simulink model "z6_backup"  (R2016b)
settings: Solver=VariableStepAuto  StartTime=0.0  StopTime=10.0  RelTol=1e-3
values from neighbouring files (symbols this model uses):
  K = acker(A, B, p)    [z6.m]    (also in z7.m; z8.m)
  x0 = [0.1 0.1 0.1]    [z3.m]    (also in z6.m = [-1 2 1]; z7.m = [0 0 0]; z8.m = [-1 2 1])
settings Model: Creator=E7440  LastModifiedBy=E7440

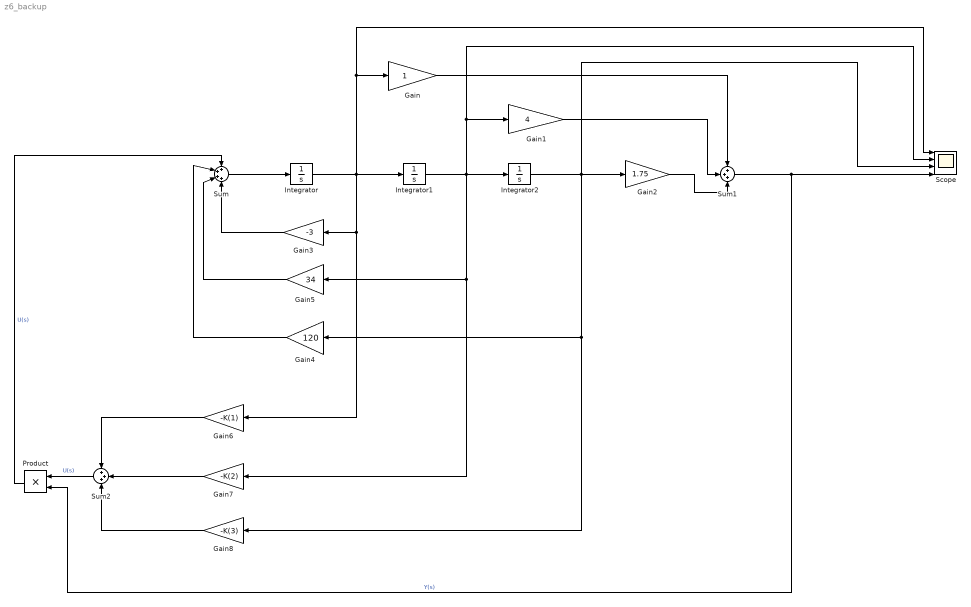
== system z6_backup ==
  Gain : Gain
  Gain1 : Gain  Gain=4
  Gain2 : Gain  Gain=1.75
  Gain3 : Gain  Gain=-3
  Gain4 : Gain  Gain=120
  Gain5 : Gain  Gain=34
  Gain6 : Gain  Gain=-K(1)
  Gain7 : Gain  Gain=-K(2)
  Gain8 : Gain  Gain=-K(3)
  Integrator : Integrator  InitialCondition=x0(1)
  Integrator1 : Integrator  InitialCondition=x0(2)
  Integrator2 : Integrator  InitialCondition=x0(3)
  Product : Product
  Scope : Scope  NumInputPorts=4
  Sum : Sum  Inputs=++++
  Sum1 : Sum  Inputs=+++
  Sum2 : Sum  Inputs=3
  wires:
  Product/1 -> Sum/1  "U(s)"
  Sum/1 -> Integrator/1
  Gain2/1 -> Sum1/3
  Gain1/1 -> Sum1/2
  Gain/1 -> Sum1/1
  Integrator2/1 -> Scope/3, Gain8/1, Gain4/1, Gain2/1
  Integrator/1 -> Integrator1/1, Gain6/1, Gain3/1, Gain/1, Scope/1
  Gain3/1 -> Sum/4
  Integrator1/1 -> Integrator2/1, Gain7/1, Gain5/1, Gain1/1, Scope/2
  Gain4/1 -> Sum/2
  Gain5/1 -> Sum/3
  Sum1/1 -> Scope/4, Product/2  "Y(s)"
  Gain7/1 -> Sum2/2
  Gain6/1 -> Sum2/1
  Gain8/1 -> Sum2/3
  Sum2/1 -> Product/1  "U(s)"
